simulink model "UART_test"  (R2024b)
settings: Solver=FixedStepAuto  StartTime=0.0  StopTime=300  FixedStep=0.01  RelTol=1e-3  EnableMultiTasking=on
libraries: arduinolib x2
settings Model: ExtModeTrigDuration=2  Creator=USER  LastModifiedBy=USER
settings SolverCC: AutoInsertRateTranBlk=on
settings OptimizationCC: EnhancedBackFolding=on  PassReuseOutputArgsAs=Individual arguments  ZeroExternalMemoryAtStartup=off  ZeroInternalMemoryAtStartup=off  MaxStackSize=64  OptimizeBlockOrder=speed  DifferentSizesBufferReuse=on  OptimizationCustomize=off  EfficientTunableParamExpr=on
settings DebuggingCC: ParameterTunabilityLossMsg=error
settings HardwareCC: ProdBitPerInt=16  ProdBitPerPointer=16  ProdBitPerSizeT=16  ProdBitPerPtrDiffT=16  ProdLargestAtomicFloat=None  ProdWordSize=8  ProdHWDeviceType=Atmel->AVR
settings SFSimCC: MATLABDynamicMemAlloc=off
settings RTWCC: Description=Embedded Coder  SystemTargetFile=ert.tlc  HardwareBoard=Arduino Mega 2560  TemplateMakefile=ert_default_tmf  Toolchain=Arduino AVR  BuildConfiguration=Faster Runs
settings CodeAppCC: ForceParamTrailComments=on  IgnoreCustomStorageClasses=off  OperatorAnnotations=on  SimulinkDataObjDesc=on  SFDataObjDesc=on  InsertBlockDesc=on
settings ERTTargetCC: SupportContinuousTime=on  SupportVariableSizeSignals=on  ExtModeTransport=3  ExtModeStaticAlloc=on  ExtModeAutomaticAllocSize=off  ExtModeStaticAllocSize=2048  ExtModeMexFile=ext_xcp  ExtModeIntrfLevel=Level2 - Open  InlinedParameterPlacement=Hierarchical

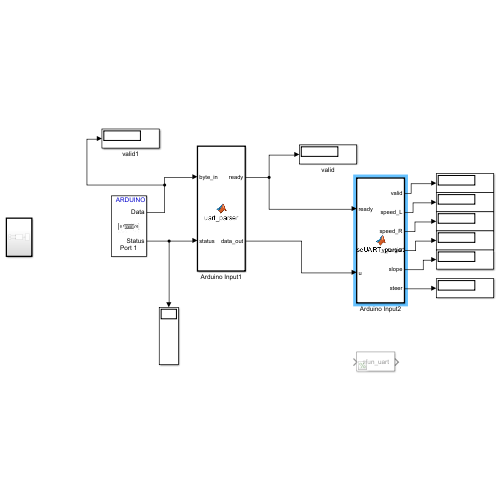
[thumbnail: Simulink's stored preview of the top-level diagram]
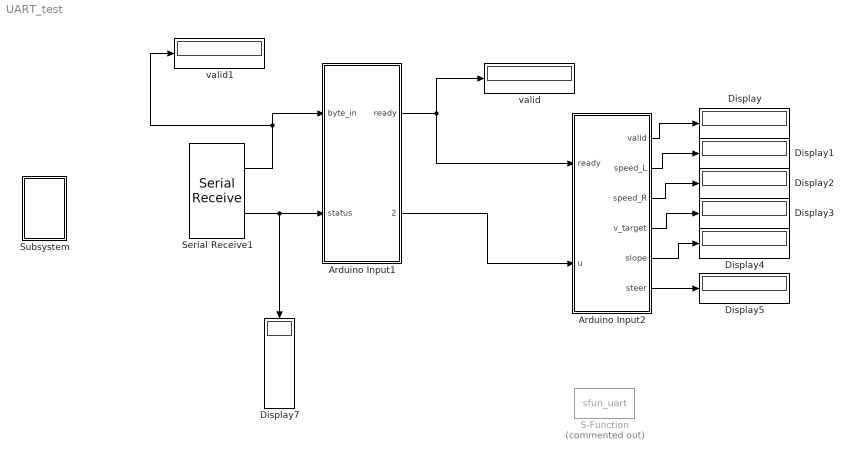
== system UART_test ==
  Arduino Input1 : MATLAB Function  TreatAsAtomicUnit=on
  Arduino Input2 : MATLAB Function  TreatAsAtomicUnit=on
  Display{,1..5,7} (7 alike) : Display
  S-Function : S-Function  Commented=on  FunctionName=sfun_uart  SFunctionDeploymentMode=off  EnableBusSupport=off
  Serial Receive1 : arduinolib/Serial Receive  portNumber=1  DataType=uint8  blockPlatform=ARDUINO  TimeOut=0  MaxDataLength=10  isARMArch=off  DataLengthOption=Length via dialog  Datalength=1  Header=[]  Terminator=[]  SampleTime=0.01  ShowOutStatus=on
      settings: SourceProductName=Common
  Subsystem : Subsystem  TreatAsAtomicUnit=on  SystemSampleTime=1
  valid : Display
  valid1 : Display
  wires:
  Arduino Input1/2(data_out) -> Arduino Input2/2(u)
  Arduino Input1/1(ready) -> valid/1, Arduino Input2/1(ready)
  Serial Receive1/1 -> valid1/1, Arduino Input1/1(byte_in)
  Serial Receive1/2 -> Display7/1, Arduino Input1/2(status)
  Arduino Input2/1(valid) -> Display/1
  Arduino Input2/2(speed_L) -> Display1/1
  Arduino Input2/3(speed_R) -> Display2/1
  Arduino Input2/4(v_target) -> Display3/1
  Arduino Input2/5(slope) -> Display4/1
  Arduino Input2/6(steer) -> Display5/1

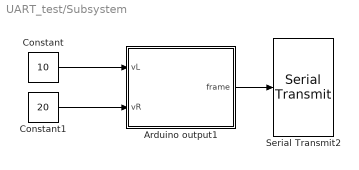
== system UART_test/Subsystem ==
  Arduino output1 : MATLAB Function  TreatAsAtomicUnit=on
  Constant : Constant  Value=10
  Constant1 : Constant  Value=20
  Serial Transmit2 : arduinolib/Serial Transmit  portNumber=1  sendmode=write  sendformat=Decimal  floatprecision=2  header=[0xAA]  terminator=[0x55]  blockPlatform=ARDUINO
      settings: SourceProductName=Common
  wires:
  Constant1/1 -> Arduino output1/2(vR)
  Arduino output1/1(frame) -> Serial Transmit2/1
  Constant/1 -> Arduino output1/1(vL)

== matlab function UART_test/Arduino Input2 ==
  data: ready input; valid output; speed_L output; speed_R output; v_target output; u input; slope output; steer output
function [valid, speed_L, speed_R, v_target, slope, steer] = parseUART_persistent(ready, u)
% UART 패킷 파서 (persistent 방식으로 이전 값 유지)
% u: [10x1] uint8, 패킷 데이터
% ready: 패킷 유효 신호

%#codegen

% 이전 출력값 저장용 persistent 변수
persistent p_valid p_speed_L p_speed_R p_v_target p_slope p_steer

% 초기화 (최초 실행 시)
if isempty(p_valid)
    p_valid = false;
    p_speed_L = 0.0;
    p_speed_R = 0.0;
    p_v_target = uint8(0);
    p_slope = uint8(0);
    p_steer = int8(0);
end

% 새로운 데이터가 들어왔을 경우만 업데이트
if ready == 1
        p_valid = true;
        p_speed_L = double(u(2));
        p_speed_R = double(u(3));
        p_v_target = u(4);
        p_slope = u(5);
        p_steer = int8(u(6));
end

% 항상 마지막 유효 출력 반환
valid     = p_valid;
speed_L   = p_speed_L;
speed_R   = p_speed_R;
v_target  = p_v_target;
slope     = p_slope;
steer     = p_steer;

== matlab function UART_test/Subsystem/Arduino output1 ==
  data: frame output; vL input; vR input
function frame = makeFrame(vL, vR)
% 입력:
%   vL, vR : 좌/우 목표 속도 (실수, cm/s 단위)
% 출력:
%   frame : 7-byte UART 전송 프레임 (uint8 벡터)
    frame = zeros(5,1,'uint8');  % 7바이트 프레임

    % 2-3. 목표속도_L (정수 + 소수)
    frame(1) = uint8(floor(vL));                       % 정수부
    frame(2) = uint8(floor(mod(vL * 100, 100)));       % 소수부 (소수점 둘째 자리까지)

    % 4-5. 목표속도_R (정수 + 소수)
    frame(3) = uint8(floor(vR));                       % 정수부
    frame(4) = uint8(floor(mod(vR * 100, 100)));       % 소수부

    % 6. CRC: 256 - (sum of byte 1~5) % 256
    crc = mod(sum(double(frame(1:5))), 256);
    frame(5) = uint8(mod(256 - crc, 256));
    
end

== matlab function UART_test/Arduino Input1 ==
  data: ready output; data_out output; byte_in input; status input
function [ready, data_out] = uart_parser(byte_in, status)
% UART 프레임 수신기 (Start Byte = 0xAA, Total = 10 bytes)
% 입력: byte_in - 1바이트씩 들어오는 uint8
% 입력: status - Serial Receive의 상태 (1이면 수신 성공)
% 출력: ready - 1이면 패킷 파싱 완료
% 출력: data_out - [1x10] uint8, 패킷 데이터

persistent buffer count collecting

if isempty(buffer)
    buffer = zeros(1, 8, 'uint8');
    count = 0;
    collecting = false;
end

ready = false;
data_out = zeros(1,8,'uint8');

if status == 1
    if ~collecting
        % 아직 수집 시작 전 → start byte 찾기
        if byte_in == hex2dec('AA')
            buffer(1) = byte_in;
            count = 1;
            collecting = true;
        end
    else
        % 수집 중
        count = count + 1;
        buffer(count) = byte_in;

        if count == 8
            data_out = buffer;
            ready = true;
            count = 0;
            collecting = false;
        end
    end
end
